simulink model "QAM"  (R2021a)
settings: Solver=VariableStepAuto  StartTime=0.0  StopTime=0.005  RelTol=1e-3
libraries: commsrccod2 x6, dspsigops x4, dsparch4 x3, commchan3 x2, commrandsrc3 x2, commsink2 x1, dspindex x1, commdigbbndam3 x1
settings Model: Creator=MrCai  LastModifiedBy=MrCai

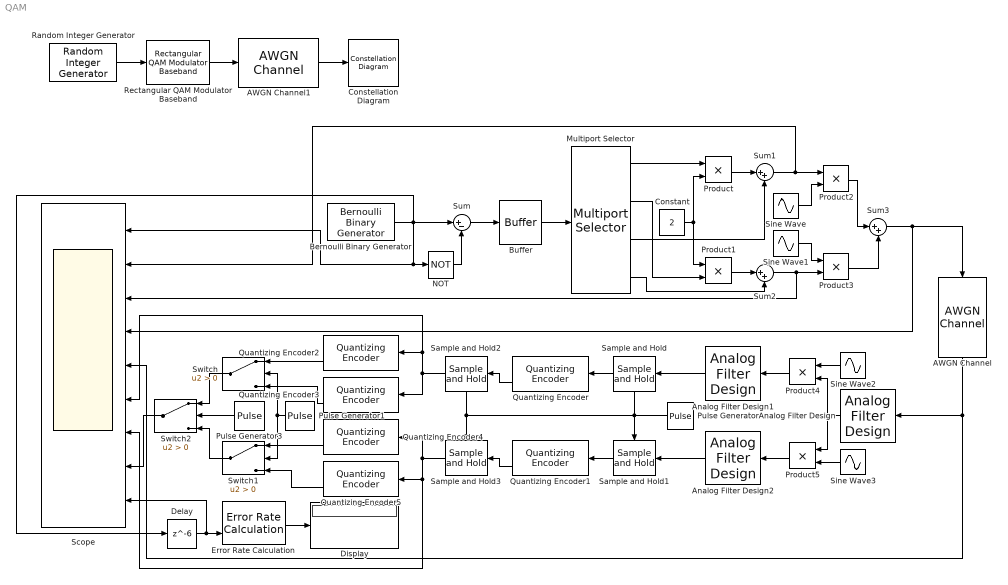
== system QAM ==
  AWGN Channel : commchan3/AWGN Channel  InputProcessing=Columns as channels (frame based)  seed=67  noiseMode="Signal to noise ratio  (SNR)"  EbNodB=10  EsNodB=10  SNRdB=30  bitsPerSym=1  Ps=1  Tsym=1  variance=1
  AWGN Channel1 : commchan3/AWGN Channel  InputProcessing=Columns as channels (frame based)  seed=67  noiseMode="Signal to noise ratio  (SNR)"  EbNodB=10  EsNodB=10  SNRdB=10  bitsPerSym=1  Ps=1  Tsym=1  variance=1
  Analog Filter Design : dsparch4/Analog Filter Design  method=Butterworth  filttype=Bandpass  N=8  Wlo=2*pi*90*1000  Whi=2*pi*110*1000  Rp=2  Rs=40
  Analog Filter Design1 : dsparch4/Analog Filter Design  method=Butterworth  filttype=Lowpass  N=8  Wlo=2*pi*10*1000  Whi=80  Rp=2  Rs=40
  Analog Filter Design2 : dsparch4/Analog Filter Design  method=Butterworth  filttype=Lowpass  N=8  Wlo=2*pi*10*1000  Whi=80  Rp=2  Rs=40
  Bernoulli Binary Generator : commrandsrc3/Bernoulli Binary Generator  ProbabilityOfZero=0.5  SeedSource=Auto  Seed=0  SampleTime=1/10000  SamplesPerFrame=1  OutputDataType=double  SimulateUsing=Interpreted execution
  Buffer : Buffer  N=4  OutputFrames=off
  Constant : Constant  Value=2
  Constellation Diagram : ConstellationDiagram
  Delay : Delay  DelayLength=6
  Display : Display
  Error Rate Calculation : commsink2/Error Rate Calculation  N=0  st_delay=6  cp_mode=Entire frame  subframe=[]  PMode=Port  WsName=ErrorVec  RsMode2=off  stop=off  numErr=100  maxBits=1e6
  Multiport Selector : dspindex/Multiport Selector  rowsOrCols=Rows  idxCellArray={1,2,3,4}  idxErrMode=Clip Index
  NOT : Logic  Operator=NOT  IconShape=distinctive  AllPortsSameDT=off  OutDataTypeStr=boolean
  Product{,1..5} (6 alike) : Product
  Pulse Generator : DiscretePulseGenerator  PhaseDelay=6  SampleTime=1/10000
  Pulse Generator1 : DiscretePulseGenerator  Period=4  PulseWidth=2  PhaseDelay=6  SampleTime=1/10000
  Pulse Generator3 : DiscretePulseGenerator  SampleTime=1/10000
  Quantizing Encoder : commsrccod2/Quantizing Encoder  partition=[-1.9 0 1.9]  codebook=[-3 -1 1 3]  idxDType=double
      settings: SourceProductBaseCode=CM
  Quantizing Encoder1 : commsrccod2/Quantizing Encoder  partition=[-1.9 0 1.9]  codebook=[-3 -1 1 3]  idxDType=double
      settings: SourceProductBaseCode=CM
  Quantizing Encoder2 : commsrccod2/Quantizing Encoder  partition=[-2 0 2]  codebook=[0 0 1 1]  idxDType=double
      settings: SourceProductBaseCode=CM
  Quantizing Encoder3 : commsrccod2/Quantizing Encoder  partition=[-2 0 2]  codebook=[0 1 0 1]  idxDType=double
      settings: SourceProductBaseCode=CM
  Quantizing Encoder4 : commsrccod2/Quantizing Encoder  partition=[-2 0 2]  codebook=[0 0 1 1]  idxDType=double
      settings: SourceProductBaseCode=CM
  Quantizing Encoder5 : commsrccod2/Quantizing Encoder  partition=[-2 0 2]  codebook=[0 1 0 1]  idxDType=double
      settings: SourceProductBaseCode=CM
  Random Integer Generator : commrandsrc3/Random Integer Generator  SetSize=16  SeedSource=Auto  Seed=0  SampleTime=1/10000  SamplesPerFrame=1  OutputDataType=double  SimulateUsing=Interpreted execution
  Rectangular QAM Modulator Baseband : commdigbbndam3/Rectangular QAM Modulator Baseband  M=16  InType=Integer  Enc=Gray  Mapping=[0:15]  PowType=Min. distance between symbols  MinDist=0.63  AvgPow=1  PeakPow=1  Ph=0  outDtype=double  outWordLen=16  outUDDataType=sfix(16)  outFracLenMode=Best precision  outFracLen=15  outDataTypeStr=double  outLastDataTypeStr=double
  Sample and Hold{,1..3} (4 alike) : dspsigops/Sample and Hold  trig=Rising edge  initCond=0  latchinput=off
  Scope : Scope  NumInputPorts=9
  Sine Wave : Sin  Frequency=2*pi*100*1000  Phase=pi/2  SampleTime=1/1000000
  Sine Wave1 : Sin  Frequency=2*pi*100*1000  Phase=pi  SampleTime=1/1000000
  Sine Wave2 : Sin  Amplitude=2  Frequency=2*pi*100*1000  Phase=pi/2  SampleTime=1/1000000
  Sine Wave3 : Sin  Amplitude=2  Frequency=2*pi*100*1000  Phase=pi  SampleTime=1/1000000
  Sum : Sum  Inputs=|+-
  Sum1 : Sum  Inputs=|++
  Sum2 : Sum  Inputs=|++
  Sum3 : Sum  Inputs=|++
  Switch : Switch  Criteria=u2 > Threshold
  Switch1 : Switch  Criteria=u2 > Threshold
  Switch2 : Switch  Criteria=u2 > Threshold
  wires:
  Bernoulli Binary Generator/1 -> Scope/1, NOT/1, Delay/1, Sum/1
  NOT/1 -> Sum/2
  Sum/1 -> Buffer/1
  Buffer/1 -> Multiport Selector/1
  Multiport Selector/1 -> Product/1
  Constant/1 -> Product1/1, Product/2
  Product/1 -> Sum1/1
  Multiport Selector/4 -> Sum2/2
  Product1/1 -> Sum2/1
  Sum1/1 -> Scope/2, Product2/1
  Sum2/1 -> Scope/3, Product3/2
  Sine Wave1/1 -> Product3/1
  Sine Wave/1 -> Product2/2
  Product2/1 -> Sum3/1
  Product3/1 -> Sum3/2
  Sum3/1 -> AWGN Channel/1, Scope/4
  AWGN Channel/1 -> Analog Filter Design/1, Scope/5
  Sine Wave2/1 -> Product4/1
  Sine Wave3/1 -> Product5/2
  Product4/1 -> Analog Filter Design1/1
  Product5/1 -> Analog Filter Design2/1
  Analog Filter Design/1 -> Product5/1, Product4/2
  Analog Filter Design2/1 -> Sample and Hold1/1
  Analog Filter Design1/1 -> Sample and Hold/1
  Pulse Generator/1 -> Sample and Hold3/Trigger, Sample and Hold2/Trigger, Sample and Hold/Trigger, Sample and Hold1/Trigger
  Sample and Hold/1 -> Quantizing Encoder/1
  Sample and Hold1/1 -> Quantizing Encoder1/1
  Quantizing Encoder1/2 -> Sample and Hold3/1
  Quantizing Encoder/2 -> Sample and Hold2/1
  Sample and Hold2/1 -> Scope/6, Quantizing Encoder2/1, Quantizing Encoder3/1
  Sample and Hold3/1 -> Scope/7, Quantizing Encoder5/1, Quantizing Encoder4/1
  Quantizing Encoder2/2 -> Switch/1
  Quantizing Encoder3/2 -> Switch/3
  Quantizing Encoder4/2 -> Switch1/1
  Quantizing Encoder5/2 -> Switch1/3
  Switch/1 -> Switch2/1
  Switch1/1 -> Switch2/3
  Pulse Generator1/1 -> Switch1/2, Switch/2
  Multiport Selector/3 -> Sum1/2
  Multiport Selector/2 -> Product1/2
  Error Rate Calculation/1 -> Display/1
  Pulse Generator3/1 -> Switch2/2
  Delay/1 -> Scope/9, Error Rate Calculation/2
  Switch2/1 -> Scope/8
  Random Integer Generator/1 -> Rectangular QAM Modulator Baseband/1
  Rectangular QAM Modulator Baseband/1 -> AWGN Channel1/1
  AWGN Channel1/1 -> Constellation Diagram/1
